simulink model "ex_1"  (R2018b)
settings: Solver=VariableStepAuto  StartTime=0.0  StopTime=10.0  RelTol=1e-3
values from neighbouring files (symbols this model uses):
  B = 12    [mass_spring.m]
  F = 8    [mass_spring.m]
  K = 16    [mass_spring.m]
  M = 2    [mass_spring.m]
  x0 = 4    [mass_spring.m]
settings Model: Creator=student  LastModifiedBy=student

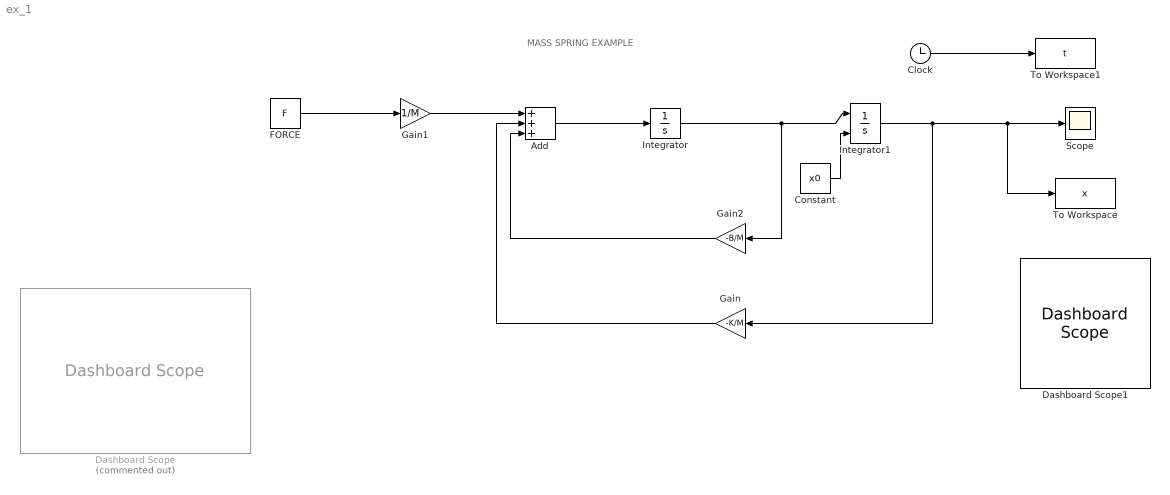
== system ex_1 ==
  note: MASS SPRING EXAMPLE
  Add : Sum  Inputs=+++
  Clock : Clock
  Constant : Constant  Value=x0
  Dashboard Scope : DashboardScope  Commented=on  WebBlockId=11
  Dashboard Scope1 : DashboardScope  WebBlockId=12
  FORCE : Constant  Value=F
  Gain : Gain  Gain=-K/M
  Gain1 : Gain  Gain=1/M
  Gain2 : Gain  Gain=-B/M
  Integrator : Integrator
  Integrator1 : Integrator  InitialConditionSource=external
  Scope : Scope
  To Workspace : ToWorkspace  VariableName=x  SampleTime=-1
  To Workspace1 : ToWorkspace  VariableName=t  SampleTime=-1
  wires:
  Integrator/1 -> Gain2/1, Integrator1/1
  Integrator1/1 -> Gain/1, To Workspace/1, Scope/1
  Add/1 -> Integrator/1
  Gain1/1 -> Add/1
  FORCE/1 -> Gain1/1
  Gain2/1 -> Add/3
  Gain/1 -> Add/2
  Clock/1 -> To Workspace1/1
  Constant/1 -> Integrator1/2
